simulink model "z_gen"  (Simulink 3.00)
settings: Solver=ode45  StartTime=0.0  StopTime=sum(inter)  RelTol=1e-3
undefined symbols (not defined in the file or in its folder): inter

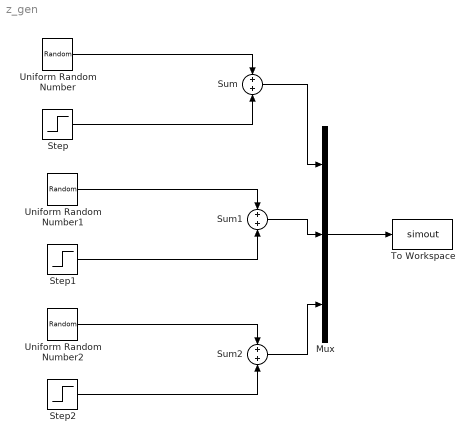
== system z_gen ==
  Mux : Mux  Inputs=3
  Step : Step  Time=inter(1)  Before=0  After=0.5  SampleTime=0
  Step1 : Step  Time=inter(2)  Before=0  After=0.5  SampleTime=0
  Step2 : Step  Time=inter(3)  Before=0  After=0.5  SampleTime=0
  Sum : Sum  Inputs=+|+  SaturateOnIntegerOverflow=on
  Sum1 : Sum  Inputs=+|+  SaturateOnIntegerOverflow=on
  Sum2 : Sum  Inputs=+|+  SaturateOnIntegerOverflow=on
  To Workspace : ToWorkspace  VariableName=simout  SampleTime=1  SaveFormat=Matrix
  Uniform Random Number : UniformRandomNumber  Minimum=0.1  Maximum=1  Seed=0  SampleTime=min(inter)/6
  Uniform Random Number1 : UniformRandomNumber  Minimum=0.5  Maximum=1.5  Seed=10  SampleTime=min(inter)/2
  Uniform Random Number2 : UniformRandomNumber  Minimum=0.3  Maximum=1.3  Seed=50  SampleTime=min(inter)/4
  wires:
  Uniform Random Number/1 -> Sum/1
  Step/1 -> Sum/2
  Uniform Random Number1/1 -> Sum1/1
  Step1/1 -> Sum1/2
  Uniform Random Number2/1 -> Sum2/1
  Step2/1 -> Sum2/2
  Sum/1 -> Mux/1
  Sum1/1 -> Mux/2
  Sum2/1 -> Mux/3
  Mux/1 -> To Workspace/1
